simulink model "test_ZMP"  (Simulink 10.2)
settings: Solver=ode45  StartTime=0.0  StopTime=2  MaxStep=Step_Time  RelTol=1e-3  EnableMultiTasking=on
settings Model: Creator=saeed  LastModifiedBy=hosse
settings DataIOCC: LimitDataPoints=on
settings OptimizationCC: ExpressionDepthLimit=2147483647
settings DebuggingCC: SolverPrmCheckMsg=warning  StateNameClashWarn=warning  SFExecutionAtInitializationDiag=warning

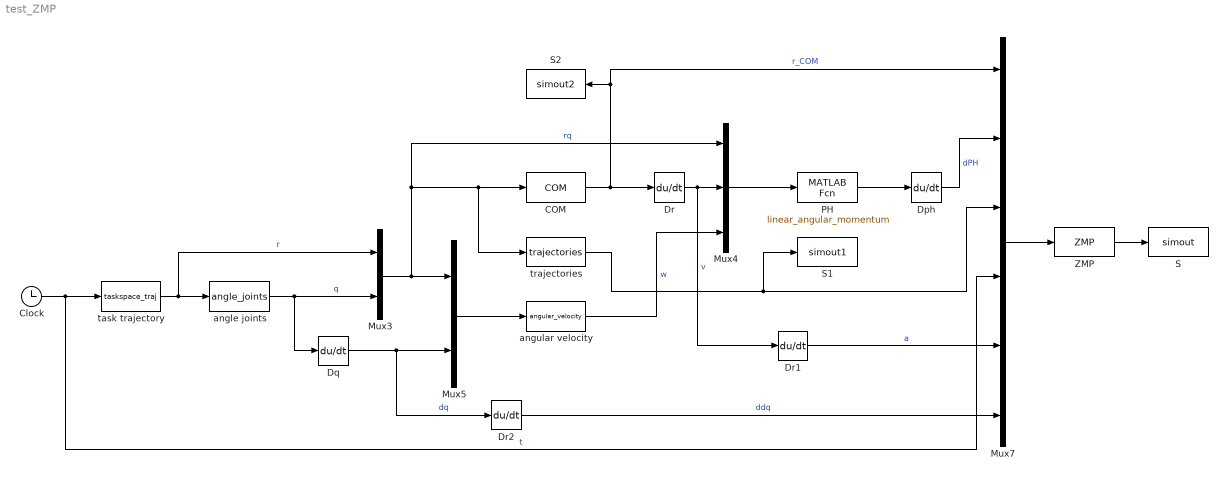
== system test_ZMP ==
  COM : MATLABFcn  MATLABFcn=COM
  Clock : Clock
  Dph : Derivative
  Dq : Derivative
  Dr : Derivative
  Dr1 : Derivative
  Dr2 : Derivative
  Mux3 : Mux  Inputs=2
  Mux4 : Mux  Inputs=3
  Mux5 : Mux  Inputs=2
  Mux7 : Mux  Inputs=6
  PH : MATLABFcn  MATLABFcn=linear_angular_momentum
  S : ToWorkspace  VariableName=simout  SaveFormat=Structure With Time  SampleTime=-1
  S1 : ToWorkspace  VariableName=simout1  SaveFormat=Structure With Time  SampleTime=-1
  S2 : ToWorkspace  VariableName=simout2  SaveFormat=Structure With Time  SampleTime=-1
  ZMP : MATLABFcn  MATLABFcn=ZMP
  angle joints : MATLABFcn  MATLABFcn=angle_joints
  angular velocity : MATLABFcn  MATLABFcn=angular_velocity
  task trajectory : MATLABFcn  MATLABFcn=taskspace_traj
  trajectories : MATLABFcn  MATLABFcn=trajectories
  wires:
  angular velocity/1 -> Mux4/3  "w"
  Clock/1 -> Mux7/4, task trajectory/1  "t"
  task trajectory/1 -> Mux3/1, angle joints/1  "r"
  angle joints/1 -> Dq/1, Mux3/2  "q"
  Mux5/1 -> angular velocity/1
  Dq/1 -> Dr2/1, Mux5/2  "dq"
  Mux3/1 -> trajectories/1, COM/1, Mux4/1, Mux5/1  "rq"
  COM/1 -> Mux7/1, S2/1, Dr/1  "r_COM"
  Dr/1 -> Dr1/1, Mux4/2  "v"
  Mux4/1 -> PH/1
  PH/1 -> Dph/1
  Dph/1 -> Mux7/2  "dPH"
  ZMP/1 -> S/1
  Mux7/1 -> ZMP/1
  trajectories/1 -> S1/1, Mux7/3
  Dr1/1 -> Mux7/5  "a"
  Dr2/1 -> Mux7/6  "ddq"
